simulink model "mcdpl"  (R2021b)
settings: Solver=VariableStepAuto  StartTime=0.0  StopTime=1e-4  RelTol=1e-3
libraries: dsparch4 x1
settings Model: Creator=zhonghuatu  LastModifiedBy=zhonghuatu

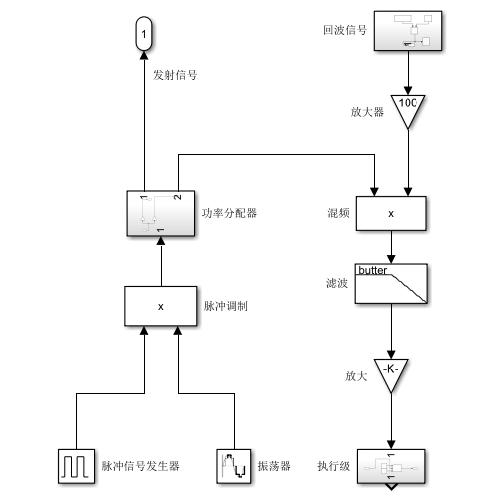
[thumbnail: Simulink's stored preview of the top-level diagram]
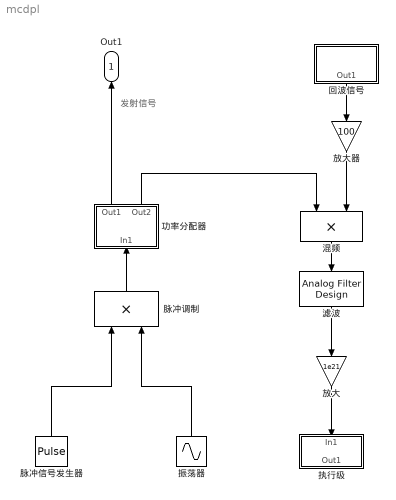
== system mcdpl ==
  note: 发射信号
  功率分配器 : Subsystem
  回波信号 : Subsystem
  执行级 : Subsystem
  振荡器 : Sin  Amplitude=100  Frequency=100e6*2*pi  Phase=10*pi/180  SampleTime=1e-10
  放大 : Gain  Gain=1e21
  放大器 : Gain  Gain=100
  混频 : Product
  滤波 : dsparch4/Analog Filter Design  method=Butterworth  filttype=Lowpass  N=8  Wlo=2.1e3  Whi=80  Rp=2  Rs=40
  脉冲信号发生器 : DiscretePulseGenerator  PulseType=Time based  Period=20e-6  PulseWidth=50  VectorParams1D=off
  脉冲调制 : Product
  Out1 : Outport
  wires:
  放大器/1 -> 混频/2
  放大/1 -> 执行级/1(In1)
  脉冲信号发生器/1 -> 脉冲调制/1
  振荡器/1 -> 脉冲调制/2
  滤波/1 -> 放大/1
  混频/1 -> 滤波/1
  脉冲调制/1 -> 功率分配器/1(In1)
  功率分配器/1(Out1) -> Out1/1
  功率分配器/2(Out2) -> 混频/1
  回波信号/1(Out1) -> 放大器/1

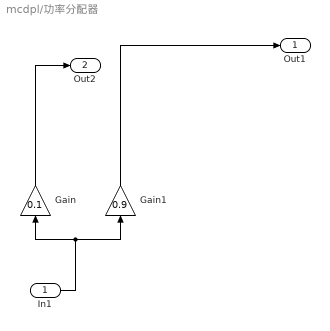
== system mcdpl/功率分配器 ==
  In1 : Inport
  Gain : Gain  Gain=0.1
  Gain1 : Gain  Gain=0.9
  Out1 : Outport
  Out2 : Outport  Port=2
  wires:
  In1/1 -> Gain1/1, Gain/1
  Gain1/1 -> Out1/1
  Gain/1 -> Out2/1

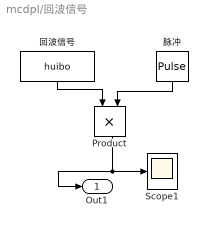
== system mcdpl/回波信号 ==
  Product : Product
  Scope1 : Scope
  回波信号 : FromWorkspace  VariableName=huibo  SampleTime=-1
  脉冲 : DiscretePulseGenerator  PulseType=Time based  Period=20e-6  PulseWidth=50  PhaseDelay=5e-6  VectorParams1D=off
  Out1 : Outport
  wires:
  脉冲/1 -> Product/2
  Product/1 -> Out1/1, Scope1/1
  回波信号/1 -> Product/1

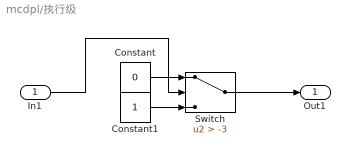
== system mcdpl/执行级 ==
  In1 : Inport
  Constant : Constant  Value=0
  Constant1 : Constant
  Switch : Switch  Criteria=u2 > Threshold  Threshold=-3
  Out1 : Outport
  wires:
  Constant1/1 -> Switch/3
  In1/1 -> Switch/2
  Constant/1 -> Switch/1
  Switch/1 -> Out1/1
